simulink model "Task6"  (R2019b)
settings: Solver=VariableStepAuto  StartTime=0.0  StopTime=10.0  RelTol=1e-3
settings Model: Creator=12393  LastModifiedBy=12393

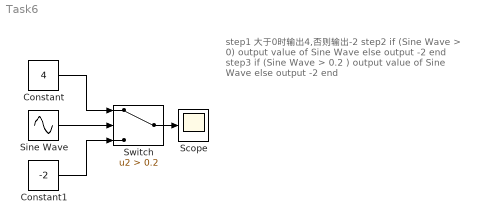
== system Task6 ==
  note: step1 大于0时输出4,否则输出-2
      | step2
      | if (Sine Wave > 0)
      | output value of Sine Wave
      | else
      | output -2
      | end
      | step3
      | if (Sine Wave > 0.2 )
      | output value of Sine Wave
      | else
      | output -2
      | end
  Constant : Constant  Value=4
  Constant1 : Constant  Value=-2
  Scope : Scope
  Sine Wave : Sin  SampleTime=0
      settings: AttributesFormatString=Frequency=%<Frequency>rad/sec
  Switch : Switch  Criteria=u2 > Threshold  Threshold=0.2
  wires:
  Sine Wave/1 -> Switch/2
  Constant/1 -> Switch/1
  Constant1/1 -> Switch/3
  Switch/1 -> Scope/1
